simulink model "lab3p2q1"  (Simulink 8.7)
settings: Solver=FixedStepDiscrete  SolverMode=SingleTasking  StartTime=0.0  StopTime=150  RelTol=1e-3
settings Model: Creator=no_alal  LastModifiedBy=no_alal
settings DataIOCC: LimitDataPoints=off  SaveFormat=Dataset
settings DebuggingCC: UnderspecifiedInitializationDetection=Simplified  MergeDetectMultiDrivingBlocksExec=error
settings HardwareCC: ProdBitPerPointer=64  ProdLargestAtomicFloat=Float  ProdIntDivRoundTo=Zero  ProdEndianess=LittleEndian  ProdWordSize=64  ProdHWDeviceType=Intel->x86-64 (Windows64)
settings ModelReferenceCC: PropagateSignalLabelsOutOfModel=on
settings ConfigComp: CovModelRefEnable=off

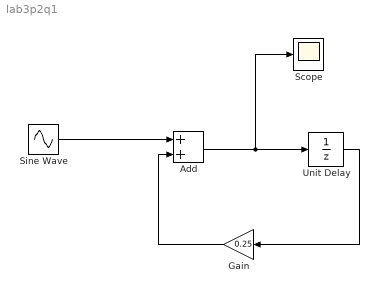
== system lab3p2q1 ==
  Add : Sum
  Gain : Gain  Gain=0.25
  Scope : Scope
  Sine Wave : Sin  Frequency=2*pi*(1/150)  SampleTime=5
  Unit Delay : UnitDelay  SampleTime=-1
  wires:
  Sine Wave/1 -> Add/1
  Add/1 -> Scope/1, Unit Delay/1
  Gain/1 -> Add/2
  Unit Delay/1 -> Gain/1
